simulink model "evse_stateflow"  (R2023b)
settings: Solver=VariableStepAuto  StartTime=0.0  StopTime=10.0  RelTol=1e-3
libraries: fl_lib x14, nesl_utility x8, ee_lib x5, simulink x2, batteryecm_lib x1
settings Model: Creator=dawid  LastModifiedBy=dawid

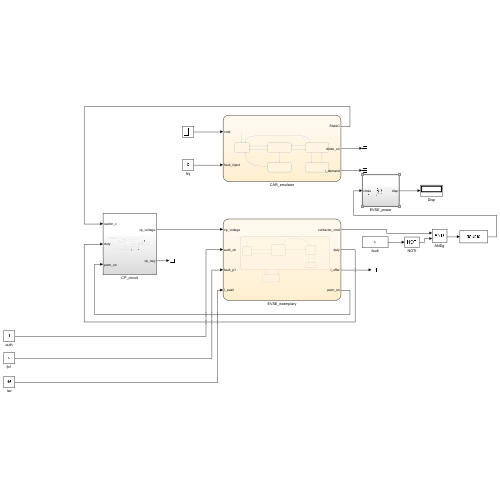
[thumbnail: Simulink's stored preview of the top-level diagram]
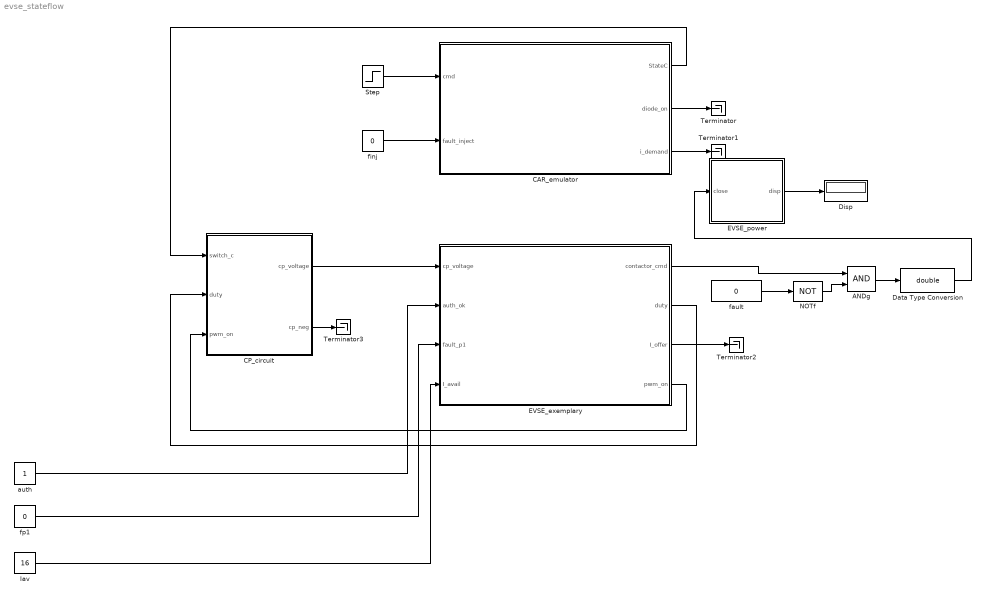
== system evse_stateflow ==
  ANDg : Logic  AllPortsSameDT=off  OutDataTypeStr=boolean
  CAR_emulator : Stateflow chart  TreatAsAtomicUnit=on
  CP_circuit : Subsystem
  Data Type Conversion : DataTypeConversion  OutDataTypeStr=double  SaturateOnIntegerOverflow=off  RndMeth=Floor
  Disp : Display
  EVSE_exemplary : Stateflow chart  TreatAsAtomicUnit=on
      settings: PortSchema="{\"entries\":[{\"content\":{\"sides\":[{\"content\":{\"connectorIds\":[\"In1\",\"In2\",\"In3\",\"In4\"]},\"type\":\"ConnectorPlacement.EquallySpacedRectSide\",\"uuid\":\"ee59908b-fb24-4855-b680-a730a874a947\"},{\"content\":{\"connectorIds\":[\"Out2\",\"Out1\",\"Out3\",\"Out4\"],\"side\":\"RIGHT\"},\"type\":\"ConnectorPlacement.EquallySpacedRectSide\",\"uuid\":\"0e5ed03d-e395-4720-8a84-1ba5b9635bf8\"},{\"content\":{\"side\":\"TOP\"},\"type\":\"ConnectorPlacement.EquallySpacedRectSide\",\"uuid\":\"a8b148f4-821f-4ab7-a7ab-1f4838aeff7c\"}]},\"type\":\"ConnectorPlacement.EquallySpacedConnector\",\"uuid\":\"e48f4ce0-11ec-46a4-b446-7e5a3d3d8087\"}],\"packageUris\":[\"http://schema.mathworks.com/mf0/Connector/R2020b\"],\"version\":\"1.0\"}"
  EVSE_power : Subsystem
  Iav : Constant  Value=16
  NOTf : Logic  Operator=NOT  AllPortsSameDT=off  OutDataTypeStr=boolean
  Step : Step  SampleTime=0
  Terminator{,1..3} (4 alike) : Terminator
  auth : Constant
  fault : Constant  Value=0
  finj : Constant  Value=0
  fp1 : Constant  Value=0
  wires:
  Iav/1 -> EVSE_exemplary/4(I_avail)
  auth/1 -> EVSE_exemplary/2(auth_ok)
  EVSE_exemplary/2(contactor_cmd) -> ANDg/1
  NOTf/1 -> ANDg/2
  ANDg/1 -> Data Type Conversion/1
  fault/1 -> NOTf/1
  CAR_emulator/2(diode_on) -> Terminator/1
  CAR_emulator/3(i_demand) -> Terminator1/1
  EVSE_exemplary/3(I_offer) -> Terminator2/1
  finj/1 -> CAR_emulator/2(fault_inject)
  Step/1 -> CAR_emulator/1(cmd)
  Data Type Conversion/1 -> EVSE_power/1(close)
  EVSE_power/1(disp) -> Disp/1
  CAR_emulator/1(StateC) -> CP_circuit/1(switch_c)
  EVSE_exemplary/1(duty) -> CP_circuit/2(duty)
  EVSE_exemplary/4(pwm_on) -> CP_circuit/3(pwm_on)
  CP_circuit/1(cp_voltage) -> EVSE_exemplary/1(cp_voltage)
  CP_circuit/2(cp_neg) -> Terminator3/1
  fp1/1 -> EVSE_exemplary/3(fault_p1)

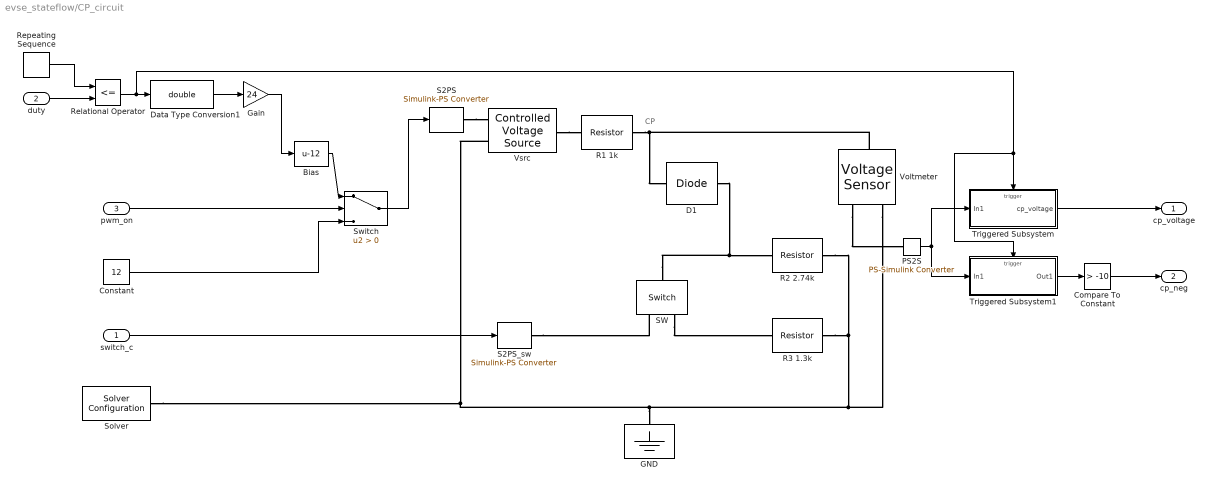
== system evse_stateflow/CP_circuit ==
  note: CP
  switch_c : Inport
  duty : Inport  Port=2
  pwm_on : Inport  Port=3
  Bias : Bias  Bias=-12  SaturateOnIntegerOverflow=off
  Compare To Constant : simulink/Logic and Bit Operations/Compare To Constant  relop=>  const=-10  OutDataTypeStr=boolean
  Constant : Constant  Value=12
  D1 : fl_lib/Electrical/Electrical Elements/Diode  Vf=0.6 V  Ron=0.3 Ohm  Goff=1e-8 1/Ohm  i_specify=off  i_priority=None  i=0 A  i_nominal_specify=off  i_nominal_unit=A  i_nominal_value=1  v_specify=off  v_priority=None  v=0 V  v_nominal_specify=off  v_nominal_unit=V  v_nominal_value=1
  Data Type Conversion1 : DataTypeConversion  OutDataTypeStr=double  SaturateOnIntegerOverflow=off  RndMeth=Floor
  GND : fl_lib/Electrical/Electrical Elements/Electrical Reference
  Gain : Gain  Gain=24
  PS2S : nesl_utility/PS-Simulink Converter  PhysicalDomain=network_engine_domain  SubClassName=ps_output  LeftPortType=input  RightPortType=output  PseudoPeriodic=off  Frequencies=[]  VectorFormat=inherit  Unit=inherit  AffineConversion=off
  R1 1k : fl_lib/Electrical/Electrical Elements/Resistor  R=1000 Ohm  i_specify=off  i_priority=None  i=0 A  i_nominal_specify=off  i_nominal_unit=A  i_nominal_value=1  v_specify=off  v_priority=None  v=0 V  v_nominal_specify=off  v_nominal_unit=V  v_nominal_value=1
  R2 2.74k : fl_lib/Electrical/Electrical Elements/Resistor  R=2740 Ohm  i_specify=off  i_priority=None  i=0 A  i_nominal_specify=off  i_nominal_unit=A  i_nominal_value=1  v_specify=off  v_priority=None  v=0 V  v_nominal_specify=off  v_nominal_unit=V  v_nominal_value=1
  R3 1.3k : fl_lib/Electrical/Electrical Elements/Resistor  R=1300 Ohm  i_specify=off  i_priority=None  i=0 A  i_nominal_specify=off  i_nominal_unit=A  i_nominal_value=1  v_specify=off  v_priority=None  v=0 V  v_nominal_specify=off  v_nominal_unit=V  v_nominal_value=1
  Relational Operator : RelationalOperator  Operator=<=  OutDataTypeStr=boolean  RndMeth=Simplest  InputSameDT=off
  Repeating Sequence : simulink/Sources/Repeating Sequence  rep_seq_t=[0 0.001]  rep_seq_y=[0 100]
  S2PS : nesl_utility/Simulink-PS Converter  PhysicalDomain=network_engine_domain  SubClassName=ps_input  LeftPortType=input  RightPortType=output  PseudoPeriodic=off  Frequencies=[]  NoiseDistribution=none  NoiseParameters=[]  Unit=1  AffineConversion=off  FilteringAndDerivatives=provide  SimscapeFilterOrder=1  InputFilterTimeConstant=0.001  UdotUserProvided=0
  S2PS_sw : nesl_utility/Simulink-PS Converter  PhysicalDomain=network_engine_domain  SubClassName=ps_input  LeftPortType=input  RightPortType=output  PseudoPeriodic=off  Frequencies=[]  NoiseDistribution=none  NoiseParameters=[]  Unit=1  AffineConversion=off  FilteringAndDerivatives=provide  SimscapeFilterOrder=1  InputFilterTimeConstant=0.001  UdotUserProvided=0
  SW : fl_lib/Electrical/Electrical Elements/Switch  R_closed=0.01 Ohm  G_open=1e-8 1/Ohm  Threshold=0.5  i_specify=off  i_priority=None  i=0 A  i_nominal_specify=off  i_nominal_unit=A  i_nominal_value=1  v_specify=off  v_priority=None  v=0 V  v_nominal_specify=off  v_nominal_unit=V  v_nominal_value=1
  Solver : nesl_utility/Solver Configuration  PhysicalDomain=network_engine_domain  SubClassName=solver  LeftPortType=input  RightPortType=generic  Tones=[]  Harmonics=[]  SimulateNoise=off  Profile=off  UseLocalSampling=off  EnableSwitchedLinearOptims=on  FrequencyDomain=off  UseCCode=off  RelTol=0.001  AbsTol=0.001  MinStep=1e-09  ToWorkspace=off  RevertToSquareIcSolve=off  NumHomotopyIterations=100  PhasorMode=off  PhasorModeNumHarmonics=1  ConsistencySolver=NEWTON_XTOL_AFTER_FTOL  IndexReductionMethod=DerivativeReplacement  DoDC=off  ResidualTolerance=1e-09  ConsistencyTolSource=GLOBAL  ConsistencyAbsTol=0.001  ConsistencyRelTol=0.001  ConsistencyTolFactor=0.001  UseLocalSolver=off  LocalSolverChoice=NE_BACKWARD_EULER_ADVANCER  ResolveIndetEquations=on  FunctionEvalNumThread=1  LocalSolverSampleTime=0.001  DoFixedCost=off  MaxNonlinIter=3  MaxModeIter=2  ComputeImpulses=off  ImpulseIterations=2  LinearAlgebra=auto  LinearAlgebraNumThread=0  EquationFormulation=NE_TIME_EF  DelaysMemoryBudget=1024  AutomaticFiltering=on  FilteringTimeConstant=0.001  PartitionStorageMethod=AS_NEEDED  PartitionMemoryBudget=1024  PartitionMethod=ROBUST  MultibodyUseLocalSolver=off  MultibodyLocalSolverChoice=ODE1  MultibodyLocalSolverSampleTime=0.001
  Switch : Switch  Criteria=u2 > Threshold  SaturateOnIntegerOverflow=off  InputSameDT=off
  Triggered Subsystem : Subsystem  TreatAsAtomicUnit=on
  Triggered Subsystem1 : Subsystem  TreatAsAtomicUnit=on
  Voltmeter : fl_lib/Electrical/Electrical Sensors/Voltage Sensor
  Vsrc : fl_lib/Electrical/Electrical Sources/Controlled Voltage Source
  cp_voltage : Outport
  cp_neg : Outport  Port=2
  wires:
  PS2S/1 -> Triggered Subsystem1/1(In1), Triggered Subsystem/1(In1)
  Triggered Subsystem1/1(Out1) -> Compare To Constant/1
  Constant/1 -> Switch/3
  Relational Operator/1 -> Triggered Subsystem1/Trigger, Triggered Subsystem/Trigger, Data Type Conversion1/1
  Compare To Constant/1 -> cp_neg/1
  Repeating Sequence/1 -> Relational Operator/1
  Gain/1 -> Bias/1
  Data Type Conversion1/1 -> Gain/1
  Switch/1 -> S2PS/1
  Bias/1 -> Switch/1
  Triggered Subsystem/1(cp_voltage) -> cp_voltage/1
  switch_c/1 -> S2PS_sw/1
  duty/1 -> Relational Operator/2
  pwm_on/1 -> Switch/2
  connections:
  S2PS/RConn1 -- Vsrc/RConn1
  GND/LConn1 -- Voltmeter/RConn2 -- R2 2.74k/RConn1 -- R3 1.3k/RConn1 -- Vsrc/RConn2 -- Solver/RConn1
  Voltmeter/RConn1 -- PS2S/LConn1
  R1 1k/RConn1 -- Voltmeter/LConn1 -- D1/LConn1
  SW/LConn1 -- D1/RConn1 -- R2 2.74k/LConn1
  S2PS_sw/RConn1 -- SW/RConn1
  Vsrc/LConn1 -- R1 1k/LConn1
  SW/RConn2 -- R3 1.3k/LConn1

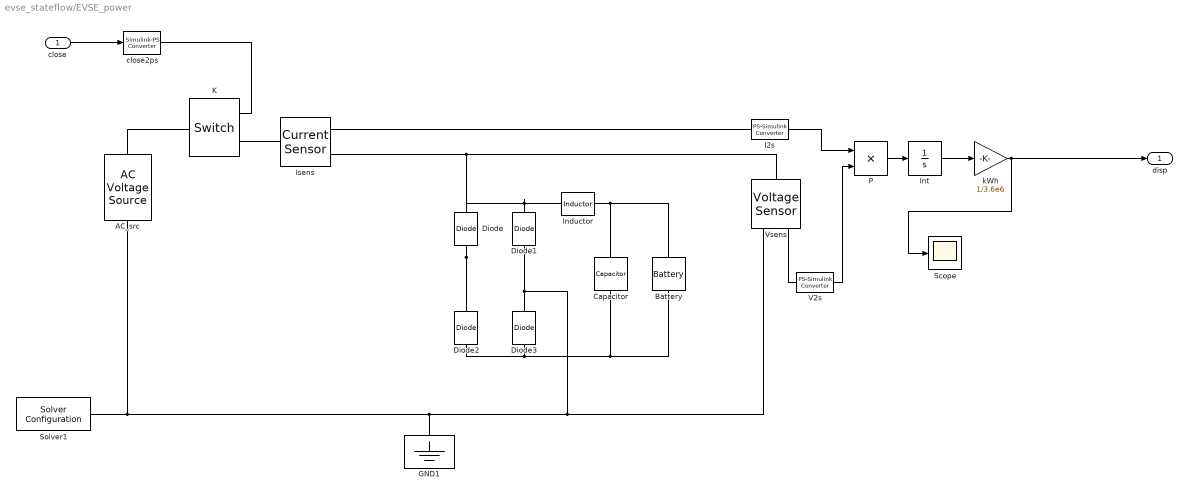
== system evse_stateflow/EVSE_power ==
  close : Inport
  AC_src : fl_lib/Electrical/Electrical Sources/AC Voltage Source  amp=325 V  shift=0 deg  frequency=50 Hz  omega=0 rad/s
  Battery : batteryecm_lib/Battery  Vnom=12 V  prm_dir=simscape.enum.battery.prm_dir.disabled  R1_dis=2 Ohm  R1_ch=2 Ohm  R1=2 Ohm  prm_AH=simscape.enum.battery.prm_AH.infinite  AH=50 A*hr  V1=11.5 V  AH1=25 A*hr  prm_R2=simscape.enum.battery.prm_R2.disabled  R2=2000 Ohm  Tmeas=298.15 K  charge_measurement_port=simscape.enum.battery.enable.no  prm_dyn=simscape.enum.battery.prm_dyn.off  Rp1=0.005 Ohm  tau1=30 s  Rp2=0.005 Ohm  tau2=30 s  Rp3=0.005 Ohm  tau3=30 s  Rp4=0.005 Ohm  tau4=30 s  Rp5=0.005 Ohm  tau5=30 s  prm_fade=simscape.enum.battery.prm_fade.disabled  N_fade=100  AH_fade=45 A*hr  R1_fade=2.02 Ohm  R1_ch_fade=2.02 Ohm  V1_fade=10.35 V  prm_age=simscape.enum.battery.prm_age.disabled  prm_age_OCV=simscape.enum.battery.prm_age_OCV.OCV  OCV_age=0.9  SOC_age=60  Tmeas_age=298.15 K  delta_time_age_vec=[0] d  temperature_age_vec=[273] K  OCV_scaling_age=2.2134e6  OCV_offset_age=1.632e6  temp_exp_age=0.515833569 V  t_exp_age=0.75  Vnom_T2=12 V  R1_T2=2.2 Ohm  R1_T2_dis=2.2 Ohm  R1_T2_ch=2.2 Ohm  V1_T2=11.4 V  R2_T2=2200 Ohm  Rp1_T2=0.005 Ohm  tau1_T2=30 s  Rp2_T2=0.005 Ohm  tau2_T2=30 s  Rp3_T2=0.005 Ohm  tau3_T2=30 s  Rp4_T2=0.005 Ohm  tau4_T2=30 s  Rp5_T2=0.005 Ohm  tau5_T2=30 s  Tmeas2=273.15 K  thermal_port=simscape.enum.thermaleffects.omit  thermal_mass=30000 J/K  i_specify=off  i_priority=None  i=0 A  i_nominal_specify=off  i_nominal_unit=A  i_nominal_value=1  v_specify=off  v_priority=None  v=0 V  v_nominal_specify=off  v_nominal_unit=V  v_nominal_value=1  charge_specify=off  charge_priority=High  charge=50 A*hr  charge_nominal_specify=off  charge_nominal_unit=A*hr  charge_nominal_value=1  num_cycles_specify=off  num_cycles_priority=High  num_cycles=0  num_cycles_nominal_specify=off  num_cycles_nominal_unit=1  num_cycles_nominal_value=1  temperature_specify=off  temperature_priority=High  temperature=298.15 K  temperature_nominal_specify=off  temperature_nominal_unit=K  temperature_nominal_value=1
  Capacitor : fl_lib/Electrical/Electrical Elements/Capacitor  c=1e-6 F  r=1e-6 Ohm  g=0 1/Ohm  i_specify=off  i_priority=None  i=0 A  i_nominal_specify=off  i_nominal_unit=A  i_nominal_value=1  v_specify=off  v_priority=None  v=0 V  v_nominal_specify=off  v_nominal_unit=V  v_nominal_value=1  vc_specify=off  vc_priority=High  vc=0 V  vc_nominal_specify=off  vc_nominal_unit=V  vc_nominal_value=1
  Diode{,1..3} (4 alike) : ee_lib/Semiconductors & Converters/Diode  ModelType=ee.enum.diode.modelType.pwl  TableType=ee.enum.diode.tableType.IfMat  IfMat=[.07, .12, .19, 1.75, 4.24, 7.32, 11.2; .16, .3, .72, 2.14, 5.02, 8.35, 13.12] A  VfMat=[.9, 1.15, 1.25, 1.5, 1.75, 2.17, 2.6, 2.85; .58, .68, .75, 1.1, 1.38, 1.77, 2.27, 2.7] V  TjVec=[25, 125] degC  VfVec=[.5, .7, .9, 1.3, 1.7, 2.1, 2.5] V  IfVec=[.1, .2, .5, 1, 2, 4, 7, 10] A  Vf=0.6 V  Ron=0.3 Ohm  Goff=1e-8 S  prmExp=ee.enum.diode.expParam.useTwo  I12=[.0137, .545] A  V12=[.6, .7] V  RS=0 Ohm  Tmeas=25 degC  IS=1e-12 A  ec=1  I1=0.0137 A  V1=0.6 V  N_series=1  N_parallel=1  ZenerEnable=false  Rz=0.3 Ohm  BV=inf V  C_param=ee.enum.diode.capParam.fixed  CJ=0 pF  CJ0=5 pF  Vvec=[.1, 10, 100] V  Cvec=[3.5, 1, .4] pF  VJ=1 V  Mgrad=0.5  FC=0.5  Q_param=ee.enum.diode.recoveryParam.off  iRM=-7.15 A  iF=4 A  didt=-750 A/us  trr_factor=3  trr=115 ns  Qrr=150 nA*s  Vr=-600 V  Ls=150 nH  Erec=0.03 J  TT=50 ns  tau=100 ns  T_param=ee.enum.diode.temperatureParam.off  Tdevice=25 degC  I1_T2=0.245 A  V1_T2=0.5 V  IS_T2=1.25e-7 A  Tmeas2=125 degC  XTI_param=ee.enum.diode.xtiParam.pn  XTI=3  EG_param=ee.enum.diode.egapParam.material_si  EG=1.11 eV  dBVdT=0 V/K  enable_faults=simscape.enum.onoff.off  fault_action=simscape.enum.assert.action.none  fault_types=ee.enum.diode.faults.open  tau_fault=1e-3 s  IfMat_faulted=[.07, .12, .19, 1.75, 4.24, 7.32, 11.2; .16, .3, .72, 2.14, 4.02, 6.35, 9.12] A  VfMat_faulted=[.9, 1.15, 1.25, 1.5, 1.75, 2.17, 2.6, 2.85; .58, .68, .75, 1.1, 1.38, 1.77, 2.27, 2.7] V  VfVec_faulted=[.5, .7, .9, 1.3, 1.7, 2.1, 2.5] V  IfVec_faulted=[.1, .2, .5, 1, 2, 4, 7, 10] A  Ropen_faulted=1000 Ohm  Gshort_faulted=1000 1/Ohm  Vf_faulted=0.6 V  Ron_faulted=0.3 Ohm  Goff_faulted=1e-8 S  I12_faulted=[.0137, .545] A  V12_faulted=[.6, .7] V  IS_faulted=1e-12 A  ec_faulted=1  I1_faulted=0.0137 A  V1_faulted=0.6 V  RS_faulted=0 Ohm  Rz_faulted=0.3 Ohm  BV_faulted=inf V  Cscale_faulted=100  fault_trigger=ee.enum.faults.faultTrigger.temporal  t_fault=inf s  max_permissible_voltage=inf V  n_fail_on_voltage=1  max_permissible_current=inf A  t_fail_on_current=1 s  max_permissible_dVdt=inf V/s  enable_fault_input=simscape.enum.onoff.off  i_specify=off  i_priority=None  i=0 A  i_nominal_specify=off  i_nominal_unit=A  i_nominal_value=1  v_specify=off  v_priority=None  v=0 V  v_nominal_specify=off  v_nominal_unit=V  v_nominal_value=1  v_capacitor_specify=off  v_capacitor_priority=None  v_capacitor=0 V  v_capacitor_nominal_specify=off  v_capacitor_nominal_unit=V  v_capacitor_nominal_value=1  faulted_specify=off  faulted_priority=None  faulted=0  faulted_nominal_specify=off  faulted_nominal_unit=1  faulted_nominal_value=1  i_diode_specify=off  i_diode_priority=None  i_diode=0 A  i_diode_nominal_specify=off  i_diode_nominal_unit=A  i_diode_nominal_value=1  v_diode_specify=off  v_diode_priority=None  v_diode=0 V  v_diode_nominal_specify=off  v_diode_nominal_unit=V  v_diode_nominal_value=1  i_capacitor_specify=off  i_capacitor_priority=None  i_capacitor=0 A  i_capacitor_nominal_specify=off  i_capacitor_nominal_unit=A  i_capacitor_nominal_value=1  power_dissipated_specify=off  power_dissipated_priority=None  power_dissipated=0 W  power_dissipated_nominal_specify=off  power_dissipated_nominal_unit=W  power_dissipated_nominal_value=1  fidelity_level=ee.enum.diode.fidelity.includeChargeDyn  rec_loss_model=ee.enum.diode.reverseRecoveryModel.fixed  ErecVal=0 J  scaleWithIandV=true  ErecMat=zeros(2, 3) J  TjrecVec=[298.15, 398.15] K  IfrecVec=[.1, 1, 10] A  IrecVal=10 A  VrecVal=10 V  tFilter=1 / 1000 / 100 s  max_permissible_temperature=inf K  t_fail_on_temperature=1 s  thermal_network_parameterization=ee.enum.thermalNetworkTopology.junctionCase  Rth=[0, 10] K/W  Rth_Cauer=[1, 3, 10] K/W  Rth_Foster=[4, 6] K/W  thermal_mass_parameterization=ee.enum.thermalNetwork.timeconstant  thermal_mass=[0, 1] J/K  thermal_mass_Cauer=[.1, .3, 1] J/K  thermal_mass_Foster=[1.5, 3] J/K  thermal_time_constant=[0, 10] s  thermal_time_constant_Cauer=[1, 3, 10] s  thermal_time_constant_Foster=[6, 18] s  thermal_mass_initial_temperatures=[25, 25] degC  thermal_mass_initial_temperatures_Cauer=[25, 25, 25] degC  junction_thermal_mass=0.01 J/K  Tvec_initial_Foster=[25, 25, 25, 25] degC  no_thermal_network=0  junction_temperature_specify=off  junction_temperature_priority=None  junction_temperature=25 degC  junction_temperature_nominal_specify=off  junction_temperature_nominal_unit=degC  junction_temperature_nominal_value=1
  GND1 : fl_lib/Electrical/Electrical Elements/Electrical Reference
  I2s : nesl_utility/PS-Simulink Converter  PhysicalDomain=network_engine_domain  SubClassName=ps_output  LeftPortType=input  RightPortType=output  PseudoPeriodic=off  Frequencies=[]  VectorFormat=inherit  Unit=inherit  AffineConversion=off
  Inductor : ee_lib/Passive/Inductor  l=1e-6 H  enable_L_tol=ee.enum.toleranceApplication.none  L_tol=20  tol_distribution=ee.enum.toleranceDistribution.uniform  nSigma=4  r=0 Ohm  g=1e-9 1/Ohm  enable_operating_limits=ee.enum.enable.no  operating_limit_action=ee.enum.passive.reportOpLim.warn  max_working_current=1 A  power_rating=1 W  enable_faults=ee.enum.enable.no  fault_action=simscape.enum.assert.action.none  lambdaPercent=50  k_faulted=0.9999  turnsShort=ee.enum.passive.inductor.turnsShortOption.no  openCct=ee.enum.enable.no  groundShort=ee.enum.passive.inductor.groundShortOption.no  groundShortG=0 1/Ohm  tau_fault=1e-3 s  fault_trigger=ee.enum.faults.faultTrigger.temporal  t_fault=1 s  max_permissible_voltage=100 V  n_fail_on_voltage=1  max_permissible_current=1 A  t_fail_on_current=1 s  i_L_specify=off  i_L_priority=High  i_L=0 A  i_L_nominal_specify=off  i_L_nominal_unit=A  i_L_nominal_value=1
  Int : Integrator
  Isens : fl_lib/Electrical/Electrical Sensors/Current Sensor
  K : fl_lib/Electrical/Electrical Elements/Switch  R_closed=0.01 Ohm  G_open=1e-8 1/Ohm  Threshold=0.5  i_specify=off  i_priority=None  i=0 A  i_nominal_specify=off  i_nominal_unit=A  i_nominal_value=1  v_specify=off  v_priority=None  v=0 V  v_nominal_specify=off  v_nominal_unit=V  v_nominal_value=1
  P : Product
  Scope : Scope
  Solver1 : nesl_utility/Solver Configuration  PhysicalDomain=network_engine_domain  SubClassName=solver  LeftPortType=input  RightPortType=generic  Tones=[]  Harmonics=[]  SimulateNoise=off  Profile=off  UseLocalSampling=off  EnableSwitchedLinearOptims=on  FrequencyDomain=off  UseCCode=off  RelTol=0.001  AbsTol=0.001  MinStep=1e-09  ToWorkspace=off  RevertToSquareIcSolve=off  NumHomotopyIterations=100  PhasorMode=off  PhasorModeNumHarmonics=1  ConsistencySolver=NEWTON_XTOL_AFTER_FTOL  IndexReductionMethod=DerivativeReplacement  DoDC=off  ResidualTolerance=1e-09  ConsistencyTolSource=GLOBAL  ConsistencyAbsTol=0.001  ConsistencyRelTol=0.001  ConsistencyTolFactor=0.001  UseLocalSolver=off  LocalSolverChoice=NE_BACKWARD_EULER_ADVANCER  ResolveIndetEquations=on  FunctionEvalNumThread=1  LocalSolverSampleTime=0.001  DoFixedCost=off  MaxNonlinIter=3  MaxModeIter=2  ComputeImpulses=off  ImpulseIterations=2  LinearAlgebra=auto  LinearAlgebraNumThread=0  EquationFormulation=NE_TIME_EF  DelaysMemoryBudget=1024  AutomaticFiltering=on  FilteringTimeConstant=0.001  PartitionStorageMethod=AS_NEEDED  PartitionMemoryBudget=1024  PartitionMethod=ROBUST  MultibodyUseLocalSolver=off  MultibodyLocalSolverChoice=ODE1  MultibodyLocalSolverSampleTime=0.001
  V2s : nesl_utility/PS-Simulink Converter  PhysicalDomain=network_engine_domain  SubClassName=ps_output  LeftPortType=input  RightPortType=output  PseudoPeriodic=off  Frequencies=[]  VectorFormat=inherit  Unit=inherit  AffineConversion=off
  Vsens : fl_lib/Electrical/Electrical Sensors/Voltage Sensor
  close2ps : nesl_utility/Simulink-PS Converter  PhysicalDomain=network_engine_domain  SubClassName=ps_input  LeftPortType=input  RightPortType=output  PseudoPeriodic=off  Frequencies=[]  NoiseDistribution=none  NoiseParameters=[]  Unit=1  AffineConversion=off  FilteringAndDerivatives=provide  SimscapeFilterOrder=1  InputFilterTimeConstant=0.001  UdotUserProvided=0
  kWh : Gain  Gain=1/3.6e6
  disp : Outport
  wires:
  Int/1 -> kWh/1
  P/1 -> Int/1
  kWh/1 -> disp/1, Scope/1
  I2s/1 -> P/1
  V2s/1 -> P/2
  close/1 -> close2ps/1
  connections:
  K/RConn2 -- Isens/LConn1
  Vsens/RConn1 -- V2s/LConn1
  AC_src/RConn1 -- K/LConn1
  Isens/RConn1 -- I2s/LConn1
  close2ps/RConn1 -- K/RConn1
  Solver1/RConn1 -- AC_src/LConn1 -- Diode3/RConn1 -- Diode1/LConn1 -- Vsens/RConn2 -- GND1/LConn1
  Capacitor/LConn1 -- Battery/LConn1 -- Inductor/RConn1
  Diode1/RConn1 -- Diode/RConn1 -- Inductor/LConn1
  Capacitor/RConn1 -- Battery/RConn1 -- Diode2/LConn1 -- Diode3/LConn1
  Diode2/RConn1 -- Isens/RConn2 -- Vsens/LConn1 -- Diode/LConn1

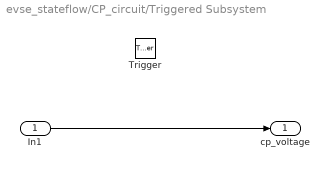
== system evse_stateflow/CP_circuit/Triggered Subsystem ==
  In1 : Inport
  Trigger : TriggerPort  TriggerType=falling  VariantControl=(inherit)
  cp_voltage : Outport
  wires:
  In1/1 -> cp_voltage/1

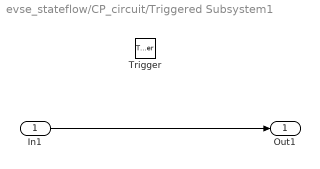
== system evse_stateflow/CP_circuit/Triggered Subsystem1 ==
  In1 : Inport
  Trigger : TriggerPort  VariantControl=(inherit)
  Out1 : Outport
  wires:
  In1/1 -> Out1/1

== stateflow chart evse_stateflow/EVSE_exemplary ==
  note: Petla 3 (aplikacja): auth_ok, I_avail = nastawy/limity (RFID, DLB, harmonogram).
  state Operating
    state Detected
      entry: pwm_on=1;
      I_offer=I_avail;
      duty=I_offer/0.6;
      contactor_cmd=0;
    state Charging
      entry: contactor_cmd=1;
      during: I_offer=I_avail;
      duty=I_offer/0.6;
    state Idle
      entry: pwm_on=0;
      duty=0;
      contactor_cmd=0;
      I_offer=0;
    state Ventilation
      entry: contactor_cmd=1;
    Charging -> Detected [order 1] : [cp_voltage>7.5 && cp_voltage<10.5]
    (default) -> Idle
    Idle -> Detected : [cp_voltage>7.5 && cp_voltage<10.5]
    Detected -> Charging [order 1] : [cp_voltage>4.5 && cp_voltage<7.5 && auth_ok==1]
    Detected -> Idle [order 2] : [cp_voltage>10.5]
    Charging -> Ventilation [order 2] : [cp_voltage>1.5 && cp_voltage<4.5]
    Ventilation -> Charging : [cp_voltage>4.5 && cp_voltage<7.5]
  state Tripped
    entry: contactor_cmd=0; pwm_on=0; duty=0;
  note: Petla 1 (bezpieczenstwo): fault_p1 = OR(RCD, PE, zwarcie CP, sklejenie). Weto nadrzedne.
  note: I_offer/duty: duty=I_offer/0.6 (10-85%). DLB: during w Charging sledzi I_avail.
  (default) -> Operating
  Tripped -> Operating : [fault_p1==0]
  Operating -> Tripped : [fault_p1==1]
  data: cp_voltage input; auth_ok input; fault_p1 input; I_avail input; duty output; contactor_cmd output; I_offer output; pwm_on output

== stateflow chart evse_stateflow/CAR_emulator ==
  note: Emulator auta: pasywny elektrycznie - wybiera rezystory/diode.
  state A_Unplugged
    entry: diode_on=0;
    StateC=0;
    i_demand=0;
  state B_Connected
    entry: diode_on=1;
    StateC=0;
    i_demand=0;
  state C_Ready
    entry: StateC=1;
    i_demand=16;
  state Fault
    entry: diode_on=0;
    StateC=0;
    i_demand=0;
  state D_Ventilation
    entry: StateC=1;
    i_demand=10;
  (default) -> A_Unplugged
  C_Ready -> A_Unplugged [order 3] : [cmd==0]
  C_Ready -> B_Connected [order 1] : [cmd==3]
  A_Unplugged -> B_Connected : [cmd==1]
  B_Connected -> C_Ready [order 1] : [cmd==2]
  B_Connected -> A_Unplugged [order 2] : [cmd==0]
  Fault -> A_Unplugged : [fault_inject==0]
  B_Connected -> Fault [order 3] : [fault_inject==1]
  C_Ready -> D_Ventilation [order 2] : [cmd==4]
  D_Ventilation -> C_Ready : [cmd==2]
  data: cmd input; fault_inject input; StateC output; diode_on output; i_demand output
